simulink model "Two_Mass_Spring_Damper_System"  (R2022a)
settings: Solver=VariableStepAuto  StartTime=0.0  StopTime=20  RelTol=1e-3
settings Model: Creator=ersad  LastModifiedBy=ersad

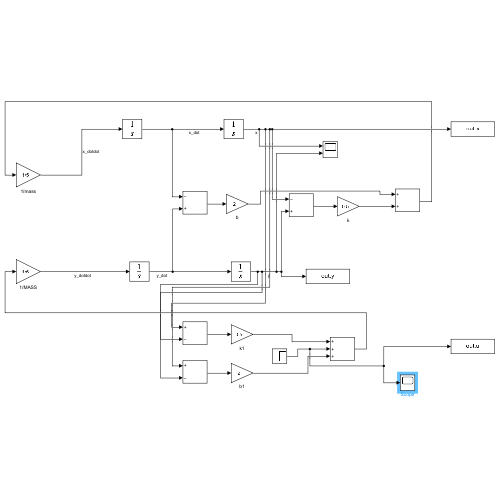
[thumbnail: Simulink's stored preview of the top-level diagram]
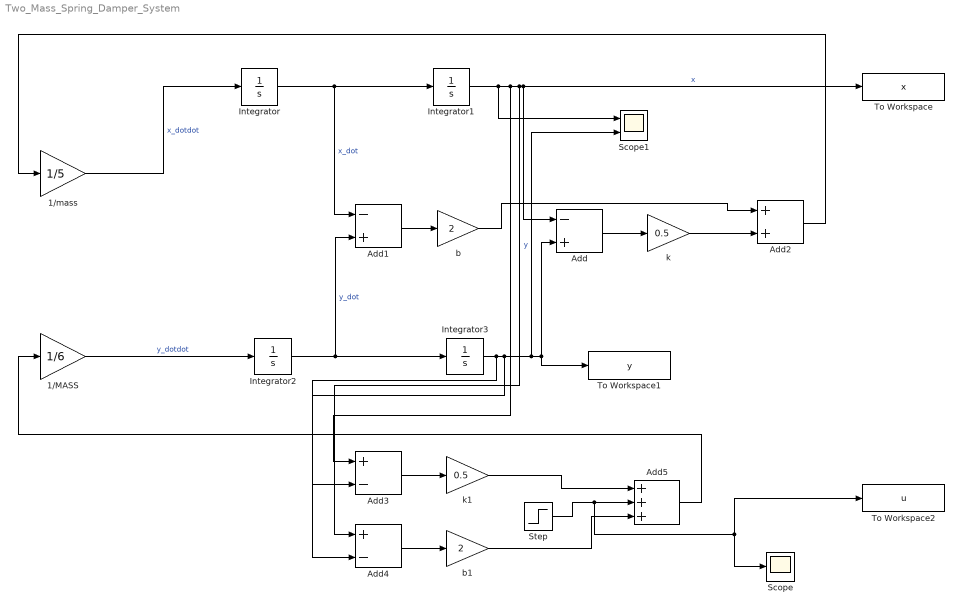
== system Two_Mass_Spring_Damper_System ==
  1/MASS : Gain  Gain=1/6
  1/mass : Gain  Gain=1/5
  Add : Sum  Inputs=-+
  Add1 : Sum  Inputs=-+
  Add2 : Sum
  Add3 : Sum  Inputs=+-
  Add4 : Sum  Inputs=+-
  Add5 : Sum  Inputs=+++
  Integrator{,1..3} (4 alike) : Integrator
  Scope : Scope
  Scope1 : Scope  NumInputPorts=2
  Step : Step  SampleTime=0
  To Workspace : ToWorkspace  VariableName=x  SampleTime=-1
      settings: Save2DSignal=2-D array (concatenate along first dimension)
  To Workspace1 : ToWorkspace  VariableName=y  SampleTime=-1
      settings: Save2DSignal=2-D array (concatenate along first dimension)
  To Workspace2 : ToWorkspace  VariableName=u  SampleTime=-1
      settings: Save2DSignal=2-D array (concatenate along first dimension)
  b : Gain  Gain=2
  b1 : Gain  Gain=2
  k : Gain  Gain=0.5
  k1 : Gain  Gain=0.5
  wires:
  1/mass/1 -> Integrator/1  "x_dotdot"
  Integrator/1 -> Add1/1, Integrator1/1  "x_dot"
  Integrator1/1 -> To Workspace/1, Add/1, Add4/1, Add3/1, Scope1/1  "x"
  1/MASS/1 -> Integrator2/1  "y_dotdot"
  Integrator2/1 -> Integrator3/1, Add1/2  "y_dot"
  Integrator3/1 -> Add4/2, Add3/2, To Workspace1/1, Add/2, Scope1/2  "y"
  Add/1 -> k/1
  Add1/1 -> b/1
  b/1 -> Add2/1
  k/1 -> Add2/2
  Add2/1 -> 1/mass/1
  Add3/1 -> k1/1
  Add4/1 -> b1/1
  k1/1 -> Add5/1
  b1/1 -> Add5/3
  Add5/1 -> 1/MASS/1
  Step/1 -> Scope/1, To Workspace2/1, Add5/2
